simulink model "NonLinModelMracScaled_ESO"  (R2023b)
settings: Solver=ode4  StartTime=0.0  StopTime=200  FixedStep=1e-3  RelTol=1e-3
undefined symbols (not defined in the file): Ac, AEFF, Am_bar, B_bar_mA, B_E, Bm_bar_mm, C_T, Cip, g0, k, K, Kc, Kq, L_hat_IC, L_hat_max, L_hat_min, M, M_hat_IC, M_hat_max, M_hat_min, P_bar, P_return, PA_IC, PA_Pa, PB_Pa, Ps_supply, r_v_mPs, V01, V02, V_DEAD, xc_dot_IC, xc_IC, xc_m, zm_IC
libraries: simulink x3
(part 2 of 2)

== matlab function NonLinModelMracScaled_ESO/EKF_Healthy_RealDataTuned/EKF_Discrete ==
  data: u_perc input; x_hat_out output; y_k input; Fd_est output; Qd_est output
function [x_hat_out, Fd_est, Qd_est] = sdre_6state_crio(u_perc, y_k)
%SDRE_6STATE_CRIO  Discrete 6-state Extended State Observer (ESO)
%  Fully Physical Formulation: A(x) contains internal dynamics.
%  f(x,u) contains physical flows and hard friction nonlinearities.
%  Includes x5 (Mismatched Mech Disturbance) and x6 (Matched Hyd Disturbance).
%
%  States:  x = [pos(m), vel(m/s), PA(Pa), PB(Pa), Fd(N), Qd(m^3/s)]
%  Inputs:  u_k   - valve spool displacement command [m] (max 25e-5)
%           y_k   - [pos_m; PA_Pa; PB_Pa]  (measurements)
%           Ps_k  - supply pressure [Pa]
%           Pr_k  - return pressure [Pa]
%  Outputs: x_hat_out - [pos; vel; PA; PB; Fd; Qd] state estimate
%           Fd_est    - Estimated mechanical load/friction mismatch [N]
%           Qd_est    - Estimated hydraulic internal leakage/valve mismatch [m^3/s]
%#codegen

%% ── PERSISTENT STATE ─────────────────────────────────────────────────────
persistent x_hat P_k initialized;

%% ── SYSTEM PARAMETERS ────────────────────────────────────────────────────
M       = 3.4;
d_p     = 34e-3;   
d_r     = 30e-3;
A_c     = pi/4*(d_p^2 - d_r^2);   
V_dead  = 1.5315e-5;
V_0     = A_c*(190.16e-3/2) + V_dead;   
C_t     = 3.9933e-13;
beta    = 1.6e9;
Ps_k    = 200e5; 
Pr_k    = 4e5; 

% Valve Parameters
K_sv    = 3.34e-6;
k_sv    = 1.82709080;
x0_S    = 0.46e-3;
x0_R    = 0.64e-3;
K_tare  = 2.345e-9; 
u_k     = u_perc * 25e-5; % Scale % to 25mA
% Observer design
dt          = 1e-3;
alpha_Fd    = 1;   % Mechanical disturbance decay factor
alpha_Qd    = 0.2;    % Hydraulic disturbance decay factor

% Tuning Matrices (Optimized for robust model-measurement balance)
% Q_d6 = diag([1E-12,... %x1
%              1E-5,... %x2
%              1E0, 1E0, ... %x3 x4
%              1E-7, ... %Fd
%              1e-3]); %Qd

% Q_d6: x5 serbest bırakıldı, x2 esnetildi
% Q_d6: Kinematiği katılaştırıp, x5'i öğrenmeye açıyoruz
q5 = 15; 
q6 = 1; 
Q_d6 = diag([1E-14, ... % x1: dx1/dt = x2 ilişkisi KUSURSUZ kabul edilsin (Titremeyi bu önler)
             5E-5,  ... % x2: Hızın tepe noktalarına çıkış izni
             1E0,   ... % x3: PA
             1E0,   ... % x4: PB
             q5,  ... % x5: Fd_est ÇOK hızlı güncellensin (Asimetrik sürtünmeyi anında öğrensin) % 1.5e-2 idi
             q6]);... % x6: Qd_est % 1e-3 idi

% Tuning Matrices (Optimized for robust model-measurement balance)
% Q_d6 = diag([1E-12,... %x1
%              1E-6,... %x2
%              1E0, 1E0, ... %x3 x4
%              1E-3, ... %Fd
%              1e-3]); %Qd

R_m6 = diag([1E-10, 5E-2, 5E-2]);

% Scaling (Qd is ~1e-5 m^3/s, so we scale by 1e5 to keep it ~1.0)
SC6  = [1; 1; 1e-7; 1e-7; 1e-2; 1e5];
SCI6 = [1; 1; 1e7;  1e7;  1e2;  1e-5]; % <--- Son eleman 1e-5 OLMAK ZORUNDA
I6   = eye(6);
C_sc6 = [1 0 0 0 0 0; 
         0 0 1 0 0 0; 
         0 0 0 1 0 0];

%% ── INITIALIZATION ───────────────────────────────────────────────────────
if isempty(initialized)
    % Initialize 6 states
    x_hat = [y_k(1); 0; y_k(2); y_k(3); 0; 0];
    P_k   = diag([1e-6, 1e-4, 1e-6, 1e-6, 1e-4, 1e-6]);
    initialized = true;
end

%% ── STATE EXTRACTION ────────────────────────────────────────────────────
x1 = x_hat(1); % Position
x2 = x_hat(2); % Velocity
x3 = x_hat(3); % PA
x4 = x_hat(4); % PB

%% ── STEP 1: Asymmetric Friction (Linear/Nonlinear Split) ────────────────
kv = 38;

% % A6 Matrix component (Linear Viscous Damping)
a22 = -kv / M;

F_nl = 0;



%% ── STEP 2: Robust Physical Valve Flows ─────────────────────────────────
% P_tol prevents zero derivative (inf gain) when pressure hits rails
P_tol = 0.1*1e5; % 0.1 bar tolerance


PA_c = max(Pr_k + P_tol, min(Ps_k - P_tol, x3));
PB_c = max(Pr_k + P_tol, min(Ps_k - P_tol, x4));

if u_k >= 0
    Q1_s = K_sv * sqrt(Ps_k - PA_c) * (x0_S + u_k);
    Q1_r = K_sv * sqrt(PA_c - Pr_k) * (x0_R^2 / (x0_R + k_sv*u_k));
    
    Q2_s = K_sv * sqrt(Ps_k - PB_c) * (x0_S^2 / (x0_S + k_sv*u_k)); 
    Q2_r = K_sv * sqrt(PB_c - Pr_k) * (x0_R + u_k);
else
    Q1_s = K_sv * sqrt(Ps_k - PA_c) * (x0_S^2 / (x0_S - k_sv*u_k));
    Q1_r = K_sv * sqrt(PA_c - Pr_k) * (x0_R - u_k);
    
    Q2_s = K_sv * sqrt(Ps_k - PB_c) * (x0_S - u_k);
    Q2_r = K_sv * sqrt(PB_c - Pr_k) * (x0_R^2 / (x0_R - k_sv*u_k));
end

Q1 = Q1_s - Q1_r; % Net flow into A
Q2 = Q2_s - Q2_r; % Net flow into B
% Q_return = Q1_R + Q2_R + K_tare * sqrt(Ps_k - Pr_k); 
%% ── STEP 3: State-Dependent Volumes (gamma) ─────────────────────────────
% Calculate instantaneous fluid stiffness
V_A = V_0 + A_c * x1;
V_B = V_0 - A_c * x1;

% Prevent volumes from dropping below zero geometrically
V_A = max(1e-6, V_A);
V_B = max(1e-6, V_B);

gamma_A = beta / V_A;
gamma_B = beta / V_B;

%% ── STEP 4: Build SDC Matrices (A6 and f6) ──────────────────────────────
% A6: Internal couplings and linear leakages + Disturbance Dynamics
A6 = [0,  1,               0,                 0,                0,          0;
      0,  a22,             A_c/M,            -A_c/M,            1/M,        0;
      0, -gamma_A*A_c,    -gamma_A*C_t,       gamma_A*C_t,      0,          gamma_A;
      0,  gamma_B*A_c,     gamma_B*C_t,      -gamma_B*C_t,      0,         -gamma_B;
      0,  0,               0,                 0,               -alpha_Fd,   0;
      0,  0,               0,                 0,                0,         -alpha_Qd];

% f6: External physical forces, flow inputs, and hard nonlinearities
f6 = [0;
      0;
      gamma_A * Q1;
      gamma_B * Q2; 
      0;
      0];

% Forward Euler Discrete Integration
A_d6 = I6 + dt * A6;   

%% ── STEP 5: Scale Transform ──────────────────────────────────────────────
A_d6_sc = (SC6 * SCI6') .* A_d6;   
x_sc    = SC6 .* x_hat;
f_sc    = SC6 .* f6;

%% ── STEP 6: Kalman Predict ───────────────────────────────────────────────
x_pred_sc = A_d6_sc * x_sc + dt * f_sc; 

P_pred = A_d6_sc * P_k * A_d6_sc' + Q_d6;
P_pred = 0.5*(P_pred + P_pred'); 

%% ── STEP 7: Innovation & Kalman Gain ─────────────────────────────────────
z_sc   = [SC6(1)*y_k(1); SC6(3)*y_k(2); SC6(4)*y_k(3)];
innov  = z_sc - C_sc6 * x_pred_sc;
S6     = C_sc6 * P_pred * C_sc6' + R_m6;
S6     = 0.5 * (S6 + S6');

if rcond(S6) < 1e-14
    S6 = S6 + 1e-12 * eye(3);
end

K6    = (P_pred * C_sc6') / S6;
IKH6  = I6 - K6 * C_sc6;
P_k   = IKH6 * P_pred * IKH6' + K6 * R_m6 * K6'; % Joseph Form olarak bilinir. $A P A^T + B R B^T$ y
P_k   = 0.5 * (P_k + P_k');

%% ── STEP 8: Update & Output ──────────────────────────────────────────────
x_hat = SCI6 .* (x_pred_sc + K6 * innov);

% Hard physical clamp on updated pressures
x_hat(3) = max(0, min(Ps_k, x_hat(3)));
x_hat(4) = max(0, min(Ps_k, x_hat(4)));

% Map to outputs
x_hat_out = x_hat;
Fd_est    = x_hat(5);
Qd_est    = x_hat(6);

end

== matlab function NonLinModelMracScaled_ESO/MATLAB Function ==
  data: t input; y output
function y = multisine_fcn(t)
%MULTISINE_FCN  Çok bileşenli sinüs referans sinyal üreteci
%
% Simulink MATLAB Function bloğunda kullanım:
%   Blok adı  : MultiSine
%   Giriş     : t   — Clock bloğundan [s]
%   Çıkış     : y   — Referans pozisyon [mm]
%
% Tasarım kriterleri:
%   1) PE (Persistently Exciting) — Ioannou §8.5 parametre yakınsaması
%      için en az (n_params/2) = 2 farklı frekans gerekir.
%      Burada 9 bileşen kullanıldı → güçlü PE garantisi.
%   2) Schroeder fazları → crest factor minimize edilir
%      φ_k = −π·k·(k−1)/N  →  peak/RMS ≈ √2  (tek sinüse yakın)
%   3) Yumuşak başlangıç (Hann penceresi, T_ramp=2s)
%      → t=0'da ani konum sıçraması yok, mekanik darbe yok
%   4) Amplitüd azaltma: yüksek frekans → küçük genlik
%      (hidrolik aktuatör bant genişliği kısıtı)
%
% Toplam peak tahmini (Schroeder ile): ~14 mm  (<±15 mm limit)
% RMS                                 : ~7  mm
% Crest factor                        : ~2.0
%
% Frekans aralığı: 0.5 – 12 Hz  (referans model bw: ~17 Hz)
%
% =========================================================
%  MATLAB Function bloğuna bu kodu YAPIŞTIRINkopyalayın:
%  (fonksiyon imzası dahil, yorum satırları isteğe bağlı)
% =========================================================

% ---- Bileşen tanımları ----
% Frekans [Hz]   Amplitüd [mm]
%  0.5            6.0   — quasi-static / düşük frekans
%  1.0            5.0
%  2.0            4.5
%  3.0            4.0
%  5.0            3.0   — orta bant
%  6.0            3.0   — mevcut sinüs test frekansı (doğrulama noktası)
%  8.0            2.5
% 10.0            2.0
% 12.0            1.5   — bant genişliğine yakın

N    = 9;
f_Hz = [0.5,  1.0,  2.0,  3.0,  5.0,  6.0,  8.0, 10.0, 12.0];
A_mm = [6.0,  5.0,  4.5,  4.0,  3.0,  3.0,  2.5,  2.0,  1.5];

% ---- Schroeder fazları ----
% φ_k = −π·k·(k−1)/N    k = 1..N   (1-tabanlı indis)
phi = zeros(1, N);
phi(1)  = 0.0;                             % k=1:  φ = 0
phi(2)  = -pi * 2  * 1  / N;              % k=2
phi(3)  = -pi * 3  * 2  / N;              % k=3
phi(4)  = -pi * 4  * 3  / N;              % k=4
phi(5)  = -pi * 5  * 4  / N;              % k=5
phi(6)  = -pi * 6  * 5  / N;              % k=6
phi(7)  = -pi * 7  * 6  / N;              % k=7
phi(8)  = -pi * 8  * 7  / N;              % k=8
phi(9)  = -pi * 9  * 8  / N;              % k=9

% ---- Sinyal üretimi ----
omega = 2.0 * pi * f_Hz;   % açısal frekanslar [rad/s]

y = A_mm(1) * sin(omega(1)*t + phi(1)) ...
  + A_mm(2) * sin(omega(2)*t + phi(2)) ...
  + A_mm(3) * sin(omega(3)*t + phi(3)) ...
  + A_mm(4) * sin(omega(4)*t + phi(4)) ...
  + A_mm(5) * sin(omega(5)*t + phi(5)) ...
  + A_mm(6) * sin(omega(6)*t + phi(6)) ...
  + A_mm(7) * sin(omega(7)*t + phi(7)) ...
  + A_mm(8) * sin(omega(8)*t + phi(8)) ...
  + A_mm(9) * sin(omega(9)*t + phi(9));

% ---- Yumuşak başlangıç (Hann penceresi) ----
% 0 → T_ramp saniyede tam genliğe ulaşır
% w(t) = 0.5·(1 − cos(π·t/T_ramp))   →  w(0)=0, w(T_ramp)=1
T_ramp = 2.0;   % [s]
if t < T_ramp
    w = 0.5 * (1.0 - cos(pi * t / T_ramp));
    y = y * w;
end

end

== matlab function NonLinModelMracScaled_ESO/Plant/Subsystem1/MATLAB Function ==
  data: Q1 output; Q2 output; x input; Ps input; Pr input; P1 input; P2 input; K input; k input; QR output
function [Q1, Q2, QR] = fcn(x, Ps, Pr, P1, P2, K, k)
    % x0 parametresini girişten kaldırdık, içeride asimetrik tanımlayacağız.
    
    % --- ASİMETRİK SIZINTI AYARLARI ---
    % Hedef: P_null = 70 bar (Ps=210 bar iken)
    % Bu dengeyi sağlamak için Return tarafı açıklığı daha büyük olmalı.

    % --- GÜNCELLENMİŞ ASİMETRİK SIZINTI AYARLARI ---
    % Hedef: Ps=200 bar, Pr=4.5 bar iken yaklaşık 70-75 bar denge basıncı
    % $$x_{0S} \cdot \sqrt{130} = x_{0R} \cdot \sqrt{70}$$ --> Ortalamaları
    % da bulunan x0 olacak.

    % Ortalama x0 = 0.53e-3 idi. Bunu asimetrik dağıtıyoruz:
    % x0_S = 0.47e-3;  % Supply tarafı (0.47 mA)
    % x0_R = 0.64e-3;  % Return tarafı (0.64 mA)
    
    x0_S = 0.46e-3 ;  % Supply tarafı (0.46 mA) --> bunu editledim
    x0_R = 0.64e-3 ;  % Return tarafı (0.64 mA)

    % x0_S = 0.53e-3;  % Supply tarafı (0.47 mA)
    % x0_R = 0.53e-3;  % Return tarafı (0.64 mA)

    K_tare = 2.345e-9; 
    
    % Güvenlik (Basınçlar)
    dPs1 = max(0, Ps - P1); dP1r = max(0, P1 - Pr);
    dPs2 = max(0, Ps - P2); dP2r = max(0, P2 - Pr);
    dPsr = max(0, Ps - Pr);

    if x >= 0
        % P_S -> P_1 (Supply Side - Ana Akış) -> x0_S kullan
        Q1_S = K * sqrt(dPs1) * (x0_S + x); 
        
        % P_1 -> P_R (Return Side - Sızıntı) -> x0_R kullan
        Q1_R = K * sqrt(dP1r) * (x0_R^2 / (x0_R + k*x)); 

        % P_S -> P_2 (Supply Side - Sızıntı) -> x0_S kullan
        Q2_S = K * sqrt(dPs2) * (x0_S^2 / (x0_S + k*x)); 
        
        % P_2 -> P_R (Return Side - Ana Akış) -> x0_R kullan
        Q2_R = K * sqrt(dP2r) * (x0_R + x);
    else
        % x < 0 durumu
        % Simetriyi korumak için x negatifken de Supply/Return rollerine göre
        % doğru x0'ı seçmeliyiz.
        
        % P_S -> P_1 (Supply Side - Sızıntı)
        Q1_S = K * sqrt(dPs1) * (x0_S^2 / (x0_S - k*x)); 
        
        % P_1 -> P_R (Return Side - Ana Akış)
        Q1_R = K * sqrt(dP1r) * (x0_R - x); 

        % P_S -> P_2 (Supply Side - Ana Akış)
        Q2_S = K * sqrt(dPs2) * (x0_S - x); 
        
        % P_2 -> P_R (Return Side - Sızıntı)
        Q2_R = K * sqrt(dP2r) * (x0_R^2 / (x0_R - k*x)); 
    end

    Q1 = Q1_S - Q1_R;
    Q2 = Q2_S - Q2_R;
    QR = Q1_R + (Q2_R) + K_tare * sqrt(dPsr); 
end

== matlab function NonLinModelMracScaled_ESO/Plant/Cylinder_Dynamics/Subsystem1/MATLAB Function1 ==
  data: x input; F_end output; x_dot input; xmin input; xmax input; k_end input; v_lock input
function F_end = endstop_force_simple(x, x_dot, xmin, xmax, k_end, v_lock)
%#codegen
% Very stable end-stop with velocity locking
% Minimal oscillation, solver-friendly

% v_lock : velocity below which motion is considered zero (m/s)
% Typical: 1e-3 … 5e-3

F_end = 0.0;
ccc = 1e6; 
% ---- LOWER STOP ----
if x <= xmin
    % spring force
    F_end = k_end * (xmin - x);

    % velocity lock (kill oscillation)
    if x_dot < v_lock
        F_end = F_end - ccc * x_dot;   % artificial strong damping
    end
end

% ---- UPPER STOP ----
if x >= xmax
    % spring force
    F_end = -k_end * (x - xmax);

    % velocity lock
    if x_dot > -v_lock
        F_end = F_end - ccc * x_dot;
    end
end

== matlab function NonLinModelMracScaled_ESO/Plant/Cylinder_Dynamics/Subsystem/Subsystem/MATLAB Function ==
  data: v input; F_statik output
function F_statik = fcn(v)
Fc = 18; 
Fs = 75; 
v_s = 0.016; 
C = 100; 

F_statik = Fc + (Fs - Fc)*exp(-(1*abs(v)./v_s)^2);
F_statik = F_statik * tanh(C*v);

== matlab function NonLinModelMracScaled_ESO/Plant/Cylinder_Dynamics/Friction_Simple ==
  data: v input; FF output
function FF = fcn(v)
eps_smooth = 0.1; 

% --- Pozitif Yön (v > 0) ---
kv_p = 20; kc_p = 15; ks_p = 82.9; tau_p = 0.016;

% --- Negatif Yön (v < 0) ---
kv_n = 35; kc_n = 22; ks_n = 75.17; tau_n = 0.016;

% Yumuşatılmış yön fonksiyonu (sign yerine tanh)
% Bu fonksiyon -1 ile 1 arasında yumuşak bir geçiş sağlar
smooth_sign = tanh(v ./ eps_smooth);

% Asimetrik katsayı vektörleri oluşturma
% Hızın yönüne göre katsayıları seçiyoruz
kv = (v >= 0)*kv_p + (v < 0)*kv_n;
kc = (v >= 0)*kc_p + (v < 0)*kc_n;
ks = (v >= 0)*ks_p + (v < 0)*ks_n;
tau = (v >= 0)*tau_p + (v < 0)*tau_n;

% --- Sürtünme Kuvveti Hesaplama ---
% F_viscous + F_coulomb + F_stribeck
FF = (kv .* v) + (kc .* smooth_sign) + (ks .* smooth_sign .* exp(-abs(v./tau)));

== matlab function NonLinModelMracScaled_ESO/Plant/Cylinder_Dynamics/Subsystem/Kalman_Jerk_xa ==
  settings: updateMethod=DISCRETE
  data: pos_meas input; v_est output; acc_meas input; dt input; a_est output; j_est output
function [v_est, a_est, j_est] = fcn(pos_meas, acc_meas, dt)
    % KALMAN FİLTRESİ (Jerk Augmented)
    % Durumlar: x = [Pozisyon; Hız; İvme; Jerk]
    
    % Değişkenleri hafızada tutmak için 'persistent' tanımlıyoruz
    persistent x P A H Q R I initialized
    
    % --- BAŞLANGIÇ AYARLARI (Sadece ilk adımda çalışır) ---
    if isempty(initialized)
        % Başlangıç Durumu (İlk ölçüme göre)
        x = [pos_meas; 0; acc_meas; 0]; 
        
        % Başlangıç Belirsizliği
        P = eye(4); 
        
        % Matris Tanımları (Sabitler)
        % 1. Geçiş Matrisi (Fizik: x = x0 + v*dt + 0.5*a*dt^2 + ...)
        A = [1, dt, 0.5*dt^2, (1/6)*dt^3;
             0,  1,       dt,   0.5*dt^2;
             0,  0,        1,         dt;
             0,  0,        0,          1];
         
        % 2. Ölçüm Matrisi (Sadece Pos ve Acc ölçüyoruz)
        H = [1, 0, 0, 0;
             0, 0, 1, 0];
         
        % 3. Gürültü Kovaryansları (TUNING BURADAN)
        sigma_jerk = 2000; % Sistemin vahşiliği (Spike yakalama yeteneği)
        
        % Q (Süreç Gürültüsü)
        Q = diag([dt^6/36, dt^4/4, dt^2, 1]) * sigma_jerk^2;
        
        % R (Ölçüm Gürültüsü) - Sensör güveni
        R_pos = (1e-6)^2;
        R_acc = (0.5)^2;
        R = diag([R_pos, R_acc]);
        
        I = eye(4);
        initialized = 1;
    end
    
    % --- KALMAN DÖNGÜSÜ (Her adımda çalışır) ---
    
    % 1. PREDICT (Öngörü)
    x_pred = A * x;
    P_pred = A * P * A' + Q;
    
    % 2. UPDATE (Düzeltme)
    z = [pos_meas; acc_meas]; % Ölçüm vektörü
    
    y = z - H * x_pred;       % Innovation (Hata)
    S = H * P_pred * H' + R;  % Innovation Covaryans
    K = P_pred * H' / S;      % Kalman Kazancı
    
    x = x_pred + K * y;       % Durum Güncelleme
    P = (I - K * H) * P_pred; % Kovaryans Güncelleme
    
    % 3. ÇIKTI
    v_est = x(2);
    a_est = x(3);
    j_est = x(4);
end

== matlab function NonLinModelMracScaled_ESO/Plant/Cylinder_Dynamics/Subsystem/Kalman_Jerk_xPaPb ==
  settings: updateMethod=DISCRETE
  data: j_est output; a_est output; pos_meas input; v_est output; PA input; PB input
function [j_est, a_est, v_est] = fcn(pos_meas, PA, PB)
    % PRESSURE-AIDED JERK ESTIMATOR
    % Girdiler: Pozisyon ve Basınçlar
    % Çıktı: Tertemiz Jerk (j_est)
    
    persistent x P A H Q R I initialized m AA AB
    
    % --- SABİTLER ---
    dt = 0.001;   % Örnekleme Zamanı (Simulink step size ile aynı olmalı)
    
    if isempty(initialized)
        % 1. SİSTEM TANIMLAMALARI
        m  = 3.4;       % Tahmini Hareketli Kütle (kg)
        AA = 2.0106e-04;  % A Odası Alanı (m2)
        AB = 2.0106e-04;  % B Odası Alanı (m2)
        
        % 2. DURUM VEKTÖRÜ: x = [Konum; Hız; İvme; Jerk]
        % (Sürtünme değil, doğrudan kinematiği izliyoruz)
        F_net_start = (PA*AA - PB*AB);
        a_start = F_net_start / m;
        
        x = [pos_meas; 0; a_start; 0];
        P = eye(4);
        I = eye(4);
        
        % 3. GEÇİŞ MATRİSİ (Constant Jerk Model)
        % x(k+1) = x(k) + v*dt + 0.5*a*dt^2 + 1/6*j*dt^3 ...
        A = [1, dt, 0.5*dt^2, (1/6)*dt^3;
             0,  1,       dt,   0.5*dt^2;
             0,  0,        1,         dt;
             0,  0,        0,          1];
         
        % 4. ÖLÇÜM MATRİSİ
        % z1 = Konum (x1)
        % z2 = İvme  (x3) -> Basınçtan türetilmiş "Sanal İvme"
        H = [1, 0, 0, 0;
             0, 0, 1, 0];
         
        % 5. TUNING (AYARLAR)
        % Q: Jerk ne kadar hızlı değişebilir? (Sistemin vahşiliği)
        % Yüksek değer = Zıplamaları anında yakalar (Gecikmesiz).
        sigma_jerk = 100; 
        Q = diag([dt^6/36, dt^4/4, dt^2, 1]) * sigma_jerk^2;
        
        % R: Ölçümlere ne kadar güveniyoruz?
        R_pos = (1e-6)^2; % Konum çok hassas
        R_acc = (2.0)^2;  % Basınçtan gelen ivme "gürültülüdür" (Sürtünme yok sayıldığı için)
                          % Burayı gevşek bırakıyoruz ki Kalman, konum verisiyle
                          % basınç verisini harmanlayıp doğruyu bulsun.
        R = diag([R_pos, R_acc]);
        
        initialized = 1;
    end
    
    % --- 1. SANAL İVME ÖLÇÜMÜ OLUŞTURMA ---
    % Basınç kuvvetini kütleye bölerek "Ham İvme" elde ediyoruz.
    % Not: Bu ivme sürtünmeyi içermez, bu yüzden "gürültülü/hatalı" kabul edilir.
    % Kalman bunu düzeltecek.
    F_hyd = PA * AA - PB * AB;
    a_meas_virtual = F_hyd / m; 
    
    % Ölçüm Vektörü
    z = [pos_meas; a_meas_virtual];
    
    % --- 2. KALMAN PREDICT ---
    x_pred = A * x;
    P_pred = A * P * A' + Q;
    
    % --- 3. KALMAN UPDATE ---
    y = z - H * x_pred;       % Hata (Innovation)
    S = H * P_pred * H' + R;  % Kovaryans
    K = P_pred * H' / S;      % Kazanç (Gain)
    
    x = x_pred + K * y;       % Güncelleme
    P = (I - K * H) * P_pred;
    
    % --- 4. ÇIKTILAR ---
    v_est = x(2);
    a_est = x(3);
    j_est = x(4); % İŞTE ARADIĞIN JERK!
end

== matlab function NonLinModelMracScaled_ESO/Plant/Cylinder_Dynamics/Subsystem/Subsystem1/MATLAB Function ==
  data: v input; F_statik output
function F_statik = fcn(v)
Fc = 18; 
Fs = 75; 
v_s = 0.016; 
C = 100; 

F_statik = Fc + (Fs - Fc)*exp(-(1*abs(v)./v_s)^2);
F_statik = F_statik * tanh(C*v);

== matlab function NonLinModelMracScaled_ESO/Plant/Cylinder_Dynamics/MATLAB Function1 ==
  data: v input; FF output; a input; j input
function FF = fcn(v,a,j)
% --- Geçiş Yumuşaklığı Parametresi ---
% Bu değer büyüdükçe 0'daki eğim azalır (daha eğimli geçer)
eps_smooth = 0.00223;


% --- Pozitif Yön (v > 0) ---
kv_p = 39.658; Fc_p = 25; Fs_p = 82.9; tau_p = 0.0016;

% --- Negatif Yön (v < 0) ---
kv_n = 38.5; Fc_n = 5; Fs_n = 75.17; tau_n = 0.0016;

% Yumuşatılmış yön fonksiyonu (sign yerine tanh)
% Bu fonksiyon -1 ile 1 arasında yumuşak bir geçiş sağlar
smooth_sign = tanh(v ./ eps_smooth);

% Asimetrik katsayı vektörleri oluşturma
% Hızın yönüne göre katsayıları seçiyoruz
kv = (v >= 0)*kv_p + (v < 0)*kv_n;
Fc = (v >= 0)*Fc_p + (v < 0)*Fc_n;
Fs = (v >= 0)*Fs_p + (v < 0)*Fs_n;
tau = (v >= 0)*tau_p + (v < 0)*tau_n;

F_stribeck = (kv .* v) + (Fc .* smooth_sign) + (Fs .* smooth_sign .* exp(-abs(v./tau)));

K_acc = 1.121235; 
K_jerk = 0.056481; 
kappa_delay = 0; 

FF = F_stribeck + K_acc * a  +  K_jerk*j;
